simulink model "sim_interface"  (R2019b)
settings: Solver=ode4  StartTime=0.0  StopTime=20  FixedStep=0.001  RelTol=1e-3
values from neighbouring files (symbols this model uses):
  K_AMP = 1    [NLMPC_Interface_init.m]    (also in NLMPC_LQG_Interface_init.m; init.m)
  K_EC = Pr * N_pp / ( 4 * 1024 )    (= 2.27485440932e-05)    [NLMPC_Interface_init.m]    (also in NLMPC_LQG_Interface_init.m; init.m)
  K_EP = 2 * pi / ( 4 * 1024 )    (= 0.00153398078789)    [NLMPC_Interface_init.m]    (also in NLMPC_LQG_Interface_init.m; init.m)
  KF_Ts = 0.01    [NLMPC_Interface_init.m]    (also in NLMPC_LQG_Interface_init.m; init.m)
  VMAX_AMP = 6    [NLMPC_Interface_init.m]    (also in NLMPC_LQG_Interface_init.m; init.m)
  X0 = [0 0 0 0]'    [Copy_of_NLMPC_Controlled.m]    (also in NLMPC_Controlled.m; NLMPC_Interface_init.m = [0; 0; 0; 0]; NLMPC_LQG_Interface_init.m = [0; 0; 0; 0])
  X_LIM_ENABLE = 1    [NLMPC_Interface_init.m]    (also in NLMPC_LQG_Interface_init.m; init.m)
  yref1 = [0.25 1]    [Copy_of_NLMPC_Controlled.m]    (also in NLMPC_Controlled.m = [0 1]; memoGrid.m = [-1, 1])
undefined symbols (not defined in the file or in its folder): HIL, qc_get_step_size, VMAX_DAC, X_MAX, X_MIN
libraries: quarc_library x6, simulink x1, sharedTrackingLibrary x1, mpclib x1, simulink_extras x1
settings Model: SimulationMode=external  ExtModeTrigDuration=5000  Creator=Mfotoohi  LastModifiedBy=000
settings SolverCC: PositivePriorityOrder=on
settings DataIOCC: LimitDataPoints=on  SaveFormat=Array  ReturnWorkspaceOutputs=off
settings OptimizationCC: BooleanDataType=off  ExpressionDepthLimit=2147483647  InitFltsAndDblsToZero=on  LifeSpan=inf
settings DebuggingCC: SaveWithParameterizedLinksMsg=none  UnderspecifiedInitializationDetection=Classic  MergeDetectMultiDrivingBlocksExec=none  SolverPrmCheckMsg=warning  FcnCallInpInsideContextMsg=warning  StateNameClashWarn=warning  SFUnexpectedBacktrackingDiag=warning  SFNoUnconditionalDefaultTransitionDiag=warning  SFExecutionAtInitializationDiag=none  ArithmeticOperatorsInVariantConditions=warning
settings HardwareCC: ProdBitPerPointer=32  ProdBitPerSizeT=32  ProdBitPerPtrDiffT=32  ProdLargestAtomicFloat=None  ProdIntDivRoundTo=Undefined  ProdEndianess=Unspecified  ProdWordSize=32  ProdHWDeviceType=32-bit Generic
settings ModelReferenceCC: PropagateSignalLabelsOutOfModel=off
settings SFSimCC: SimUseLocalCustomCode=off  CustomCodeUndefinedFunction=UseInterfaceOnly
settings RTWCC: Description=Quarc Win32 Target  SystemTargetFile=quarc_windows.tlc  TemplateMakefile=quarc_default_tmf  RTWUseLocalCustomCode=off
settings CodeAppCC: StateflowObjectComments=on
settings STFCustomTargetCC: TargetFcnLib=ansi_tfl_tmw.mat  TargetPreCompLibLocation=C:\PROGRA~2\QUARC\lib\2011b\windows\release  GeneratePreprocessorConditionals=Disable all  CPPClassGenCompliant=on  GRTInterface=on  SystemTargetFile=quarc_windows.tlc
settings GRTTargetCC: TargetFcnLib=ansi_tfl_tmw.mat  TargetPreCompLibLocation=C:\PROGRA~2\QUARC\lib\2011b\windows\release  TargetLangStandard=C89/C90 (ANSI)  ParMdlRefBuildCompliant=off  CompOptLevelCompliant=off  ConcurrentExecutionCompliant=off  GeneratePreprocessorConditionals=Disable all  CombineOutputUpdateFcns=off  MatFileLogging=off  GRTInterface=on  UseToolchainInfoCompliant=off  ExtMode=on  ExtModeMexFile=quarc_comm
settings ConfigComp: CovMetricSettings=dw  CovHtmlReporting=on  CovSaveCumulativeToWorkspaceVar=on  CovSaveSingleToWorkspaceVar=on  CovExternalEMLEnable=off

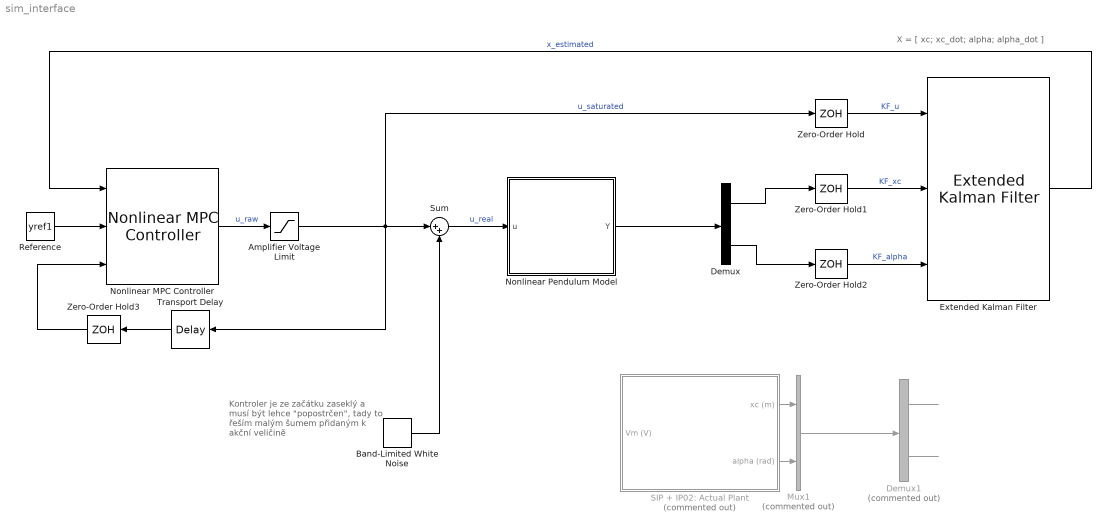
== system sim_interface ==
  note: X = [ xc; xc_dot; alpha; alpha_dot ]
  note: Kontroler je ze začátku zaseklý a musí být lehce "popostrčen", tady to řeším malým šumem přidaným k akční veličině
  Amplifier Voltage Limit : Saturate  UpperLimit=VMAX_AMP  LowerLimit=- VMAX_AMP
  Band-Limited White Noise : simulink/Sources/Band-Limited White Noise  Cov=[0.01]  Ts=0.1  seed=[23341]
  Demux : Demux  Outputs=2
  Demux1 : Demux  Commented=on  Outputs=2
  Extended Kalman Filter : sharedTrackingLibrary/Extended Kalman Filter  StateTransitionFcn=pendCartD  HasStateTransitionJacobianFcn=off  StateTransitionJacobianFcn=Jacobian  HasAdditiveProcessNoise=Additive  ProcessNoise=1  HasTimeVaryingProcessNoise=off  HasStateTransitionFcnExtraArgument=1  InitialState=X0  InitialStateCovariance=1  MeasurementFcn1=measure_x  HasMeasurementJacobianFcn1=off  HasMeasurementEnablePort1=off  HasAdditiveMeasurementNoise1=Additive  MeasurementNoise1=1  HasTimeVaryingMeasurementNoise1=off  HasMeasurementFcnExtraArgument1=0  MeasurementFcn2=measure_alpha  HasMeasurementJacobianFcn2=off  HasMeasurementEnablePort2=off  HasAdditiveMeasurementNoise2=Additive  MeasurementNoise2=1  HasTimeVaryingMeasurementNoise2=off  HasMeasurementFcnExtraArgument2=0  MeasurementFcn3=myMeasurementFcn  HasMeasurementJacobianFcn3=off  HasMeasurementEnablePort3=off  HasAdditiveMeasurementNoise3=Additive  MeasurementNoise3=1  HasTimeVaryingMeasurementNoise3=off  HasMeasurementFcnExtraArgument3=0  MeasurementFcn4=myMeasurementFcn  HasMeasurementJacobianFcn4=off  HasMeasurementEnablePort4=off  HasAdditiveMeasurementNoise4=Additive  MeasurementNoise4=1  HasTimeVaryingMeasurementNoise4=off  HasMeasurementFcnExtraArgument4=0  MeasurementFcn5=myMeasurementFcn  HasMeasurementJacobianFcn5=off  HasMeasurementEnablePort5=off  HasAdditiveMeasurementNoise5=Additive  MeasurementNoise5=1  HasTimeVaryingMeasurementNoise5=off  HasMeasurementFcnExtraArgument5=0  EnableMultirate=off  StateTransitionFcnSampleTime=1  MeasurementFcn1SampleTime=1  MeasurementFcn2SampleTime=1  MeasurementFcn3SampleTime=1  MeasurementFcn4SampleTime=1  MeasurementFcn5SampleTime=1  UseCurrentEstimator=on  OutputStateCovariance=off  DataType=double  SampleTime=KF_Ts  NumberOfMeasurements=2
      settings: SourceProductName=Automated Driving Toolbox  SourceProductBaseCode=DR
  Mux1 : Mux  Commented=on  Inputs=2
  Nonlinear MPC Controller : mpclib/Nonlinear MPC Controller  SCDEnableBlockLinearizationSpecification=on  nlmpcobj=nlobj  UseObjectTs=on  TsControl=0.1  md_enabled=off  mvtarget_enabled=off  param_enabled=off  cost_enabled=off  mvseq_enabled=off  stateseq_enabled=off  ovseq_enabled=off  slack_enabled=off  status_enabled=off  ov_min=off  ov_max=off  mv_min=off  mv_max=off  mvrate_min=off  mvrate_max=off  state_min=off  state_max=off  ov_weight=off  mv_weight=off  mvrate_weight=off  ecr_weight=off  nlp_initialize=off
      settings: SourceProductName=Model Predictive Control Toolbox
  Nonlinear Pendulum Model : Subsystem
  Reference : Constant  Value=yref1  VectorParams1D=off
  SIP + IP02: Actual Plant : Subsystem  Commented=on
  Sum : Sum  Inputs=|++
  Transport Delay : TransportDelay  DelayTime=0.01
  Zero-Order Hold : ZeroOrderHold  SampleTime=KF_Ts
  Zero-Order Hold1 : ZeroOrderHold  SampleTime=KF_Ts
  Zero-Order Hold2 : ZeroOrderHold  SampleTime=KF_Ts
  Zero-Order Hold3 : ZeroOrderHold  SampleTime=0.1
  wires:
  SIP + IP02: Actual Plant/1(xc (m)) -> Mux1/1
  SIP + IP02: Actual Plant/2(alpha (rad)) -> Mux1/2
  Nonlinear MPC Controller/1 -> Amplifier Voltage Limit/1  "u_raw"
  Amplifier Voltage Limit/1 -> Sum/1, Zero-Order Hold/1, Transport Delay/1  "u_saturated"
  Demux/1 -> Zero-Order Hold1/1
  Demux/2 -> Zero-Order Hold2/1
  Extended Kalman Filter/1 -> Nonlinear MPC Controller/1  "x_estimated"
  Transport Delay/1 -> Zero-Order Hold3/1
  Zero-Order Hold/1 -> Extended Kalman Filter/1  "KF_u"
  Zero-Order Hold1/1 -> Extended Kalman Filter/2  "KF_xc"
  Zero-Order Hold2/1 -> Extended Kalman Filter/3  "KF_alpha"
  Zero-Order Hold3/1 -> Nonlinear MPC Controller/3
  Reference/1 -> Nonlinear MPC Controller/2
  Mux1/1 -> Demux1/1
  Demux1/1 -> ?
  Demux1/2 -> ?
  Nonlinear Pendulum Model/1(Y) -> Demux/1
  Band-Limited White Noise/1 -> Sum/2
  Sum/1 -> Nonlinear Pendulum Model/1(u)  "u_real"

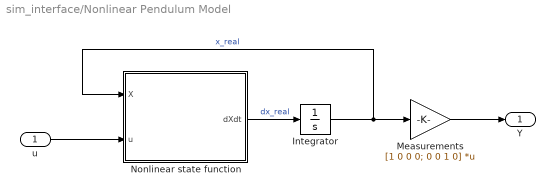
== system sim_interface/Nonlinear Pendulum Model ==
  u : Inport
  Integrator : Integrator  InitialCondition=X0
  Measurements : Gain  Gain=[1 0 0 0; 0 0 1 0]  Multiplication=Matrix(K*u)
  "Nonlinear state function " : MATLAB Function  TreatAsAtomicUnit=on
  Y : Outport
  wires:
  "Nonlinear state function "/1(dXdt) -> Integrator/1  "dx_real"
  u/1 -> "Nonlinear state function "/2(u)
  Integrator/1 -> Measurements/1, "Nonlinear state function "/1(X)  "x_real"
  Measurements/1 -> Y/1

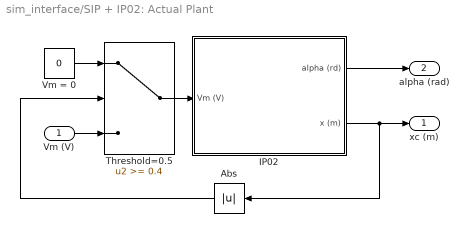
== system sim_interface/SIP + IP02: Actual Plant ==
  Vm (V) : Inport
  Abs : Abs
  "IP02 " : Subsystem
  Threshold=0.5 : Switch  Threshold=0.4  SaturateOnIntegerOverflow=on  InputSameDT=on
  Vm = 0 : Constant  Value=0
  xc (m) : Outport  InitialOutput=0
  alpha (rad) : Outport  Port=2  InitialOutput=0
  wires:
  "IP02 "/2(x (m)) -> Abs/1, xc (m)/1
  "IP02 "/1(alpha (rd)) -> alpha (rad)/1
  Threshold=0.5/1 -> "IP02 "/1(Vm (V))
  Vm = 0/1 -> Threshold=0.5/1
  Vm (V)/1 -> Threshold=0.5/3
  Abs/1 -> Threshold=0.5/2

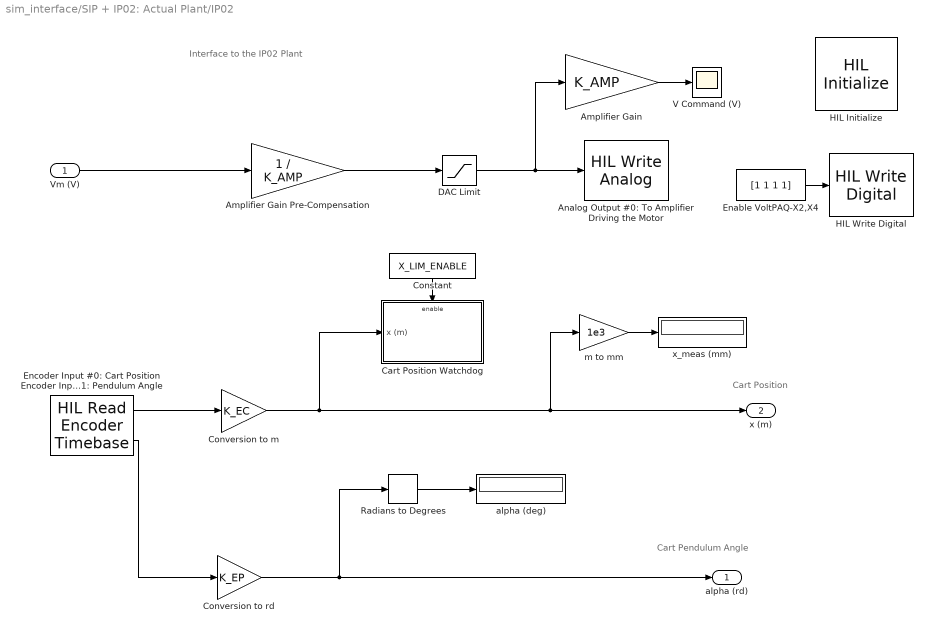
== system sim_interface/SIP + IP02: Actual Plant/IP02  ==
  note: Cart Pendulum Angle
  note: Cart Position
  note: Interface to the IP02 Plant
  Vm (V) : Inport
  Amplifier Gain : Gain  Gain=K_AMP  SaturateOnIntegerOverflow=on  OutDataTypeStr=Inherit: Same as input  ParamDataTypeStr=Inherit: Same as input
  Amplifier Gain Pre-Compensation : Gain  Gain=1 / K_AMP  SaturateOnIntegerOverflow=on  OutDataTypeStr=Inherit: Same as input  ParamDataTypeStr=Inherit: Same as input
  Analog Output #0: To Amplifier Driving the Motor : quarc_library/Data Acquisition/Generic/Immediate I//O/HIL Write Analog  Tag=unassigned  object_name=HIL-1  channels=0  sample_time=-1  active=on  vector_input=on
  Cart Position Watchdog : Subsystem  TreatAsAtomicUnit=on
  Constant : Constant  Value=X_LIM_ENABLE
  Conversion to m : Gain  Gain=K_EC  SaturateOnIntegerOverflow=on  OutDataTypeStr=Inherit: Same as input  ParamDataTypeStr=Inherit: Same as input
  Conversion to rd : Gain  Gain=K_EP  SaturateOnIntegerOverflow=on  OutDataTypeStr=Inherit: Same as input  ParamDataTypeStr=Inherit: Same as input
  DAC Limit : Saturate  UpperLimit=VMAX_DAC  LowerLimit=- VMAX_DAC
  Enable VoltPAQ-X2,X4 : Constant  Value=[1 1 1 1]
  Encoder Input #0: Cart Position Encoder Input #1: Pendulum Angle : quarc_library/Data Acquisition/Generic/Timebases/HIL Read Encoder Timebase  Tag=unassigned  object_name=HIL-1  clock=0  channels=[0 1]  samples_in_buffer=max(ceil(1/qc_get_step_size), 1)  active=on  vector_output=off  data_type_mode=Inherit via back propagation  data_type=double
  HIL Initialize : quarc_library/Data Acquisition/Generic/Configuration/HIL Initialize  object_name=HIL-1  board_type=q2_usb  board_number=0  board_options=d0=digital;d1=digital;led=auto;update_rate=normal  exclusive=off  active=off  hardware_clocks=[0:2]  clock_modes=[]  initial_clock_frequencies=[]  set_clock_params_at_start=off  set_clock_params_at_switch_in=off  set_clock_frequencies_at_start=off  set_clock_frequencies_at_switch_in=off  analog_input_channels=[0:1]  analog_input_maximums=10  analog_input_minimums=-10  set_analog_input_params_at_start=on  set_analog_input_params_at_switch_in=off  analog_output_channels=[0:1]  analog_output_maximums=10  analog_output_minimums=-10  initial_analog_outputs=[0]  final_analog_outputs=[0]  watchdog_analog_outputs=0  set_analog_output_params_at_start=on  set_analog_output_params_at_switch_in=off  set_analog_outputs_at_start=on  set_analog_outputs_at_switch_in=off  set_analog_outputs_at_terminate=on  set_analog_outputs_at_switch_out=off  set_analog_outputs_on_watchdog=off  digital_input_channels=[]  digital_output_channels=[0:7]  digital_output_configuration=[]  initial_digital_outputs=[0]  final_digital_outputs=[0]  watchdog_digital_outputs=[0]  set_digital_output_params_at_start=off  set_digital_output_params_at_switch_in=off  set_digital_outputs_at_start=on  set_digital_outputs_at_switch_in=off  set_digital_outputs_at_terminate=on  set_digital_outputs_at_switch_out=off  set_digital_outputs_on_watchdog=off  encoder_channels=[0:1]  quadrature=[4]  encoder_filter_frequency=[]  initial_encoder_counts=[0]  set_encoder_params_at_start=on  set_encoder_params_at_switch_in=off  set_encoder_counts_at_start=on  set_encoder_counts_at_switch_in=off  pwm_channels=[]  pwm_modes=[0]  pwm_frequency=1/0.020  pwm_configuration=[]  pwm_alignment=[]  pwm_polarity=[]  pwm_leading_deadband=[]  pwm_trailing_deadband=[]  initial_pwm_outputs=[0]  final_pwm_outputs=[0]  watchdog_pwm_outputs=[0]  set_pwm_params_at_start=on  set_pwm_params_at_switch_in=off  set_pwm_outputs_at_start=on  set_pwm_outputs_at_switch_in=off  set_pwm_outputs_at_terminate=on  set_pwm_outputs_at_switch_out=off  set_pwm_outputs_on_watchdog=off  other_output_channels=[]  initial_other_outputs=[]  final_other_outputs=[]  watchdog_other_outputs=[]  set_other_outputs_at_start=off  set_other_outputs_at_switch_in=off  set_other_outputs_at_terminate=off  set_other_outputs_at_switch_out=off  set_other_outputs_on_watchdog=off
  HIL Write Digital : quarc_library/Data Acquisition/Generic/Immediate I//O/HIL Write Digital  object_name=HIL-1  channels=[0:3]  sample_time=-1  active=off  vector_input=on
  Radians to Degrees : simulink_extras/Transformations/Radians to Degrees
  V Command (V) : Scope
  alpha (deg) : Display
      settings: Decimation=100
  m to mm : Gain  Gain=1e3  SaturateOnIntegerOverflow=on  OutDataTypeStr=Inherit: Same as input  ParamDataTypeStr=Inherit: Same as input
  x_meas (mm) : Display
      settings: Decimation=100
  alpha (rd) : Outport  InitialOutput=0
  x (m) : Outport  Port=2  InitialOutput=0
  wires:
  Encoder Input #0: Cart Position Encoder Input #1: Pendulum Angle/1 -> Conversion to m/1
  Conversion to m/1 -> Cart Position Watchdog/1(x (m)), x (m)/1, m to mm/1
  Amplifier Gain Pre-Compensation/1 -> DAC Limit/1
  m to mm/1 -> x_meas (mm)/1
  Encoder Input #0: Cart Position Encoder Input #1: Pendulum Angle/2 -> Conversion to rd/1
  Radians to Degrees/1 -> alpha (deg)/1
  Conversion to rd/1 -> Radians to Degrees/1, alpha (rd)/1
  Constant/1 -> Cart Position Watchdog/Enable
  DAC Limit/1 -> Analog Output #0: To Amplifier Driving the Motor/1, Amplifier Gain/1
  Vm (V)/1 -> Amplifier Gain Pre-Compensation/1
  Amplifier Gain/1 -> V Command (V)/1
  Enable VoltPAQ-X2,X4/1 -> HIL Write Digital/1

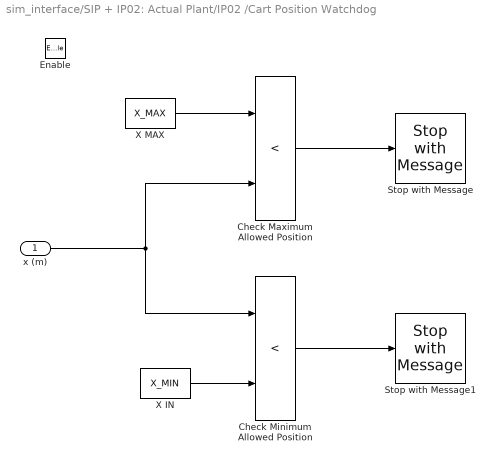
== system sim_interface/SIP + IP02: Actual Plant/IP02 /Cart Position Watchdog ==
  x (m) : Inport
  Enable : EnablePort
  Check Maximum Allowed Position : RelationalOperator  Operator=<  RndMeth=Nearest  InputSameDT=on
  Check Minimum Allowed Position : RelationalOperator  Operator=<  RndMeth=Nearest  InputSameDT=on
  Stop with Message : quarc_library/Sinks/Error Handling/Stop with Message  message_type=Fixed error message  message_icon=Error  message=Maximum Limit Reached.
  Stop with Message1 : quarc_library/Sinks/Error Handling/Stop with Message  message_type=Fixed error message  message_icon=Error  message=Minimum Limit Reached.
  X IN : Constant  Value=X_MIN
  X MAX : Constant  Value=X_MAX
  wires:
  Check Maximum Allowed Position/1 -> Stop with Message/1
  x (m)/1 -> Check Minimum Allowed Position/1, Check Maximum Allowed Position/2
  X IN/1 -> Check Minimum Allowed Position/2
  Check Minimum Allowed Position/1 -> Stop with Message1/1
  X MAX/1 -> Check Maximum Allowed Position/1

== matlab function sim_interface/Nonlinear Pendulum Model/Nonlinear state function  ==
  data: X input; u input; dXdt output
function dXdt = pendCartC(X,u)
%PENDCARTC
%    DXDT = PENDCARTC(IN1,U)

%    This function was generated by the Symbolic Math Toolbox version 8.4.
%    19-May-2020 20:15:22

X2 = X(2,:);
X3 = X(3,:);
X4 = X(4,:);
t2 = cos(X3);
t3 = sin(X3);
t4 = X4.^2;
t5 = t2.^2;
t6 = t5.*4.565807400625001e-4;
t7 = t6-3.005650706948956e-3;
t8 = 1.0./t7;
dXdt = [X2;t8.*(X2.*(-5.665253057117538e-6)+u.*5.387661376655595e-7+X4.*t2.*5.3763908601e-9+t2.*t3.*4.695776235861861e-7+t3.*t4.*1.074185854609239e-8).*(-9.53848061542277e+3);X4;t8.*(X4.*1.57714169184e-7+t3.*1.377486248645154e-5-X2.*t2.*2.524516833955624e-5+t2.*u.*2.40081805770912e-6+t2.*t3.*t4.*4.786723991704242e-8).*9.53848061542277e+3];
